simulink model "pcs_3s"  (R2025b)
settings: Solver=VariableStepAuto  StartTime=0.0  StopTime=10.0  RelTol=1e-3

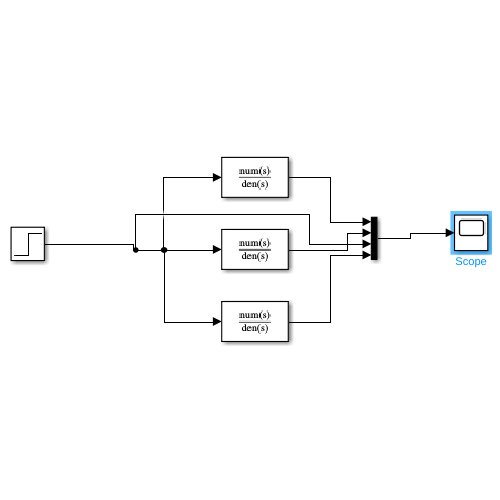
[thumbnail: Simulink's stored preview of the top-level diagram]
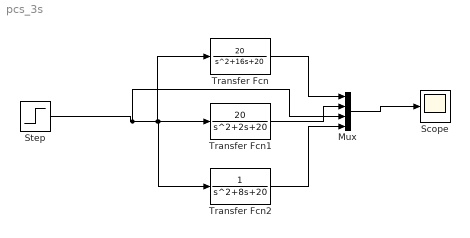
== system pcs_3s ==
  Mux : Mux
  Scope : Scope
      settings: ActiveDisplayYMinimum=-0.18567625671907279  ActiveDisplayYMaximum=1.6710863104716553
  Step : Step  Time=0  SampleTime=0
  Transfer Fcn : TransferFcn  Numerator=[20]  Denominator=[1 16 20]
  Transfer Fcn1 : TransferFcn  Numerator=[20]  Denominator=[1 2 20]
  Transfer Fcn2 : TransferFcn  Denominator=[1 8 20]
  wires:
  Transfer Fcn/1 -> Mux/1
  Transfer Fcn1/1 -> Mux/2
  Step/1 -> Mux/3, Transfer Fcn/1, Transfer Fcn2/1, Transfer Fcn1/1
  Transfer Fcn2/1 -> Mux/4
  Mux/1 -> Scope/1
